simulink model "Case4"  (R2021a)
settings: Solver=ode1  StartTime=0.0  StopTime=0.1  FixedStep=0.1e-3  RelTol=1e-3
settings Model: Creator=s.ebrahimi  LastModifiedBy=s.ebrahimi
settings DebuggingCC: AlgebraicLoopMsg=error  UnconnectedInputMsg=none  UnconnectedOutputMsg=none  UnconnectedLineMsg=none
settings ModelReferenceCC: EnableRefExpFcnMdlSchedulingChecks=off
settings RTWCC: Description=Generic Real-Time Target  GPUComputeCapability=5.0  DLArmComputeVersion=20.02.1

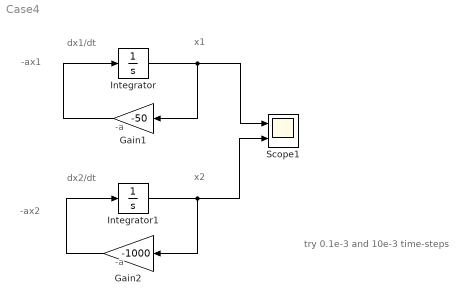
== system Case4 ==
  note: try 0.1e-3 and 10e-3 time-steps
  note: x1
  note: dx1/dt
  note: -a
  note: -ax1
  note: x2
  note: dx2/dt
  note: -a
  note: -ax2
  Gain1 : Gain  Gain=-50
  Gain2 : Gain  Gain=-1000
  Integrator : Integrator  InitialCondition=10
  Integrator1 : Integrator  InitialCondition=10
  Scope1 : Scope  NumInputPorts=2
  wires:
  Gain1/1 -> Integrator/1
  Integrator/1 -> Gain1/1, Scope1/1
  Integrator1/1 -> Scope1/2, Gain2/1
  Gain2/1 -> Integrator1/1
